simulink model "power_V2G"  (R2020b)
settings: Solver=ode23tb  StartTime=0.0  StopTime=24*60*60  RelTol=5e-4  AbsTol=5e-3
PreLoadFcn:
  | % Load Data and Parameters used by the model:
  | load power_V2G.mat
  | to=0.1;
undefined symbols (not defined in the file): A, B, C, D1, Dd, Delta, Init, j, V2G
libraries: powerlib x47, simulink x19, powerlib_meascontrol x7, simulink_extras x6, spsDieselMotorModel x1, sps_avr x1, V2Glib x1
(part 2 of 2)

== system power_V2G/Wind Farm 4.5 MW/Avoid division by zero ==
  I : Inport
  Complex to Magnitude-Angle : ComplexToMagnitudeAngle
  Magnitude-Angle to Complex : MagnitudeAngleToComplex
  Saturation1 : Saturate  UpperLimit=inf  LowerLimit=1e-6
  O : Outport  VectorParamsAs1DForOutWhenUnconnected=off
  wires:
  I/1 -> Complex to Magnitude-Angle/1
  Saturation1/1 -> Magnitude-Angle to Complex/1
  Complex to Magnitude-Angle/1 -> Saturation1/1
  Magnitude-Angle to Complex/1 -> O/1
  Complex to Magnitude-Angle/2 -> Magnitude-Angle to Complex/2

== system power_V2G/Wind Farm 4.5 MW/Break Alg. Loop 1 ==
  In : Inport
  Complex to Real-Imag : ComplexToRealImag
  Real-Imag to Complex : RealImagToComplex
  imag : Subsystem  mask(Transfer Function with Initial Outputs){N=[1], D=[to  1], Y0=0, U0=0}
      mask prompts: N "Numerator:"; D "Denominator:"; Y0 "Initial output:"; U0 "Initial input:"
      mask help: Vector expressions for numerator, and denominator. Coefficients are in descending powers of s.
      mask init:
      | [A,B,C,Dd]=tf2ss(N,D);if (isempty(Y0));[m,n]=size(A);X0=zeros(1,m); end; if (isempty(U0));[m,p]=size(B);U0=zeros(1,p);end;X0=getxo(A,B,C,Dd,U0,Y0,0);
      mask Help: Specify the initial output for the transfer function.  An optimization routine attempts to determine the appropriate initial states so that the specified initial output is achieved.  For more details, see the m-file getxo.m
      mask Display: dpoly(N,D,'s')
  real : Subsystem  mask(Transfer Function with Initial Outputs){N=[1], D=[to 1], Y0=0, U0=0}
      mask prompts: N "Numerator:"; D "Denominator:"; Y0 "Initial output:"; U0 "Initial input:"
      mask help: Vector expressions for numerator, and denominator. Coefficients are in descending powers of s.
      mask init:
      | [A,B,C,Dd]=tf2ss(N,D);if (isempty(Y0));[m,n]=size(A);X0=zeros(1,m); end; if (isempty(U0));[m,p]=size(B);U0=zeros(1,p);end;X0=getxo(A,B,C,Dd,U0,Y0,0);
      mask Help: Specify the initial output for the transfer function.  An optimization routine attempts to determine the appropriate initial states so that the specified initial output is achieved.  For more details, see the m-file getxo.m
      mask Display: dpoly(N,D,'s')
  Out : Outport  VectorParamsAs1DForOutWhenUnconnected=off
  wires:
  In/1 -> Complex to Real-Imag/1
  Real-Imag to Complex/1 -> Out/1
  real/1(Out1) -> Real-Imag to Complex/1
  imag/1(Out1) -> Real-Imag to Complex/2
  Complex to Real-Imag/2 -> imag/1(In1)
  Complex to Real-Imag/1 -> real/1(In1)

== system power_V2G/Wind Farm 4.5 MW/Wind farm control ==
  "wind " : Inport
  Compare To Constant : simulink/Logic and Bit Operations/Compare To Constant  relop=>=  const=maxwind-0.1  OutDataTypeStr=boolean  ZeroCross=off
  Compare To Constant1 : simulink/Logic and Bit Operations/Compare To Constant  relop=<=  const=nomwind  OutDataTypeStr=boolean  ZeroCross=off
  Constant1 : Constant  Value=0
  Constant2 : Constant  Value=9
  Logical Operator1 : Logic  Operator=NOT  AllPortsSameDT=off  OutDataTypeStr=boolean
  Manual Switch : ManualSwitch
  Rate Limiter2 : RateLimiter  RisingSlewLimit=1e4  FallingSlewLimit=-1e4  SampleTimeMode=inherited
  S-R Flip-Flop : simulink_extras/Flip Flops/S-R Flip-Flop  initial_condition=0
  Switch : Switch  Threshold=0.5  ZeroCross=off
  Terminator : Terminator
  Wind : Outport  VectorParamsAs1DForOutWhenUnconnected=off
  wires:
  "wind "/1 -> Switch/1, Compare To Constant/1, Compare To Constant1/1
  Constant1/1 -> Switch/3
  Logical Operator1/1 -> Switch/2
  S-R Flip-Flop/1 -> Logical Operator1/1
  Compare To Constant1/1 -> S-R Flip-Flop/2
  Compare To Constant/1 -> S-R Flip-Flop/1
  S-R Flip-Flop/2 -> Terminator/1
  Switch/1 -> Manual Switch/1
  Manual Switch/1 -> Rate Limiter2/1
  Constant2/1 -> Manual Switch/2
  Rate Limiter2/1 -> Wind/1

== system power_V2G/PV Farm 8 MW/Break Alg. Loop 1/imag ==
  In1 : Inport
  State Space : StateSpace  A=A  B=B  C=C  D=Dd  InitialCondition=X0
  Out1 : Outport  InitialOutput=0  VectorParamsAs1DForOutWhenUnconnected=off
  wires:
  State Space/1 -> Out1/1
  In1/1 -> State Space/1

== system power_V2G/PV Farm 8 MW/Break Alg. Loop 1/real ==
  In1 : Inport
  State Space : StateSpace  A=A  B=B  C=C  D=Dd  InitialCondition=X0
  Out1 : Outport  InitialOutput=0  VectorParamsAs1DForOutWhenUnconnected=off
  wires:
  State Space/1 -> Out1/1
  In1/1 -> State Space/1

== system power_V2G/Residential Load = 10 MW, PF=0.15 Industrial Load = 0.16 MVA /Residential Load/Avoid division by zero ==
  I : Inport
  Complex to Magnitude-Angle : ComplexToMagnitudeAngle
  Magnitude-Angle to Complex : MagnitudeAngleToComplex
  Saturation1 : Saturate  UpperLimit=inf  LowerLimit=1e-6
  O : Outport  VectorParamsAs1DForOutWhenUnconnected=off
  wires:
  I/1 -> Complex to Magnitude-Angle/1
  Saturation1/1 -> Magnitude-Angle to Complex/1
  Complex to Magnitude-Angle/1 -> Saturation1/1
  Magnitude-Angle to Complex/1 -> O/1
  Complex to Magnitude-Angle/2 -> Magnitude-Angle to Complex/2

== system power_V2G/Residential Load = 10 MW, PF=0.15 Industrial Load = 0.16 MVA /Residential Load/Break Alg. Loop 1 ==
  In : Inport
  Complex to Real-Imag : ComplexToRealImag
  Real-Imag to Complex : RealImagToComplex
  imag : Subsystem  mask(Transfer Function with Initial Outputs){N=[1], D=[to  1], Y0=0, U0=0}
      mask prompts: N "Numerator:"; D "Denominator:"; Y0 "Initial output:"; U0 "Initial input:"
      mask help: Vector expressions for numerator, and denominator. Coefficients are in descending powers of s.
      mask init:
      | [A,B,C,Dd]=tf2ss(N,D);if (isempty(Y0));[m,n]=size(A);X0=zeros(1,m); end; if (isempty(U0));[m,p]=size(B);U0=zeros(1,p);end;X0=getxo(A,B,C,Dd,U0,Y0,0);
      mask Help: Specify the initial output for the transfer function.  An optimization routine attempts to determine the appropriate initial states so that the specified initial output is achieved.  For more details, see the m-file getxo.m
      mask Display: dpoly(N,D,'s')
  real : Subsystem  mask(Transfer Function with Initial Outputs){N=[1], D=[to 1], Y0=0, U0=0}
      mask prompts: N "Numerator:"; D "Denominator:"; Y0 "Initial output:"; U0 "Initial input:"
      mask help: Vector expressions for numerator, and denominator. Coefficients are in descending powers of s.
      mask init:
      | [A,B,C,Dd]=tf2ss(N,D);if (isempty(Y0));[m,n]=size(A);X0=zeros(1,m); end; if (isempty(U0));[m,p]=size(B);U0=zeros(1,p);end;X0=getxo(A,B,C,Dd,U0,Y0,0);
      mask Help: Specify the initial output for the transfer function.  An optimization routine attempts to determine the appropriate initial states so that the specified initial output is achieved.  For more details, see the m-file getxo.m
      mask Display: dpoly(N,D,'s')
  Out : Outport  VectorParamsAs1DForOutWhenUnconnected=off
  wires:
  Complex to Real-Imag/1 -> real/1(In1)
  Complex to Real-Imag/2 -> imag/1(In1)
  In/1 -> Complex to Real-Imag/1
  Real-Imag to Complex/1 -> Out/1
  real/1(Out1) -> Real-Imag to Complex/1
  imag/1(Out1) -> Real-Imag to Complex/2

== system power_V2G/Residential Load = 10 MW, PF=0.15 Industrial Load = 0.16 MVA /Residential Load/Load ==
  1 : Constant
  Add : Sum
  Clock : Clock
  Constant : Constant
  Constant1 : Constant  Value=15/24
  Divide : Product  Inputs=*/
  Manual Switch : ManualSwitch
  Mux : Mux  Inputs=2
  P nom : Constant  Value=-nomPower*1e6
  Power consumption : Lookup_n-D  NumberOfTableDimensions=1  BreakpointsForDimension1=[1:timestep/60:24]  BeginIndexSearchUsingPreviousIndexResult=on  Table=datas  InternalRulePriority=Speed  RndMeth=Simplest  InputSameDT=on
  Power factor : Constant  Value=PF^2
  Product : Product
  Product1 : Product
  Scope : Scope
  Second-->Hour : Gain  Gain=1/(60*60)
  Sqrt : Sqrt  SaturateOnIntegerOverflow=on
  Sum : Sum  Inputs=-+
  PQ : Outport  VectorParamsAs1DForOutWhenUnconnected=off
  wires:
  Constant/1 -> Add/2
  1/1 -> Sum/1, Divide/1
  Second-->Hour/1 -> Add/1
  Sum/1 -> Sqrt/1
  Power factor/1 -> Divide/2
  Add/1 -> Power consumption/1
  P nom/1 -> Product/2
  Clock/1 -> Second-->Hour/1
  Sqrt/1 -> Product1/2
  Product/1 -> Product1/1, Mux/1
  Divide/1 -> Sum/2
  Product1/1 -> Mux/2
  Power consumption/1 -> Manual Switch/1
  Manual Switch/1 -> Product/1
  Constant1/1 -> Manual Switch/2
  Mux/1 -> Scope/1, PQ/1

== system power_V2G/V2G 4 MW (100x40 kW)/Car profiles/Car profile 1 ==
  Add : Sum
  Charger control : Subsystem
  Clock : Clock
  Constant : Constant
  Plug state : Lookup_n-D  NumberOfTableDimensions=1  BreakpointsForDimension1=[1:24]  BeginIndexSearchUsingPreviousIndexResult=on  Table="[1 1 1 1 1 1 0 0 1 1 1 1 1 1 1 1 0 0 1 1 1 1  1 1]"  InterpMethod=Flat  InternalRulePriority=Speed  RndMeth=Simplest  InputSameDT=on
  Rate Limiter : RateLimiter  RisingSlewLimit=1e4  FallingSlewLimit=-1e4  SampleTimeMode=inherited
  Rate Limiter1 : RateLimiter  RisingSlewLimit=1e4  FallingSlewLimit=-1e4  SampleTimeMode=inherited
  SOC initialization : Lookup_n-D  NumberOfTableDimensions=1  BreakpointsForDimension1=[1:24]  BeginIndexSearchUsingPreviousIndexResult=on  Table=[0.9 0.9 0.9 0.9 0.9 0.9 -1 0.8 0.8 0.9 0.9 0.9 0.9 0.9 0.9 0.9 -1 0.8 0.8 0.9 0.9 0.9 0.9 0.9]  InterpMethod=Flat  InternalRulePriority=Speed  RndMeth=Simplest  InputSameDT=on
  Second-->Hour : Gain  Gain=1/(60*60)
  State of charge : Subsystem
  "Regulation mode " : Outport  VectorParamsAs1DForOutWhenUnconnected=off
  "Charge mode " : Outport  Port=2  VectorParamsAs1DForOutWhenUnconnected=off
  wires:
  Constant/1 -> Add/2
  Second-->Hour/1 -> Add/1
  Clock/1 -> Second-->Hour/1
  Add/1 -> SOC initialization/1, Plug state/1
  State of charge/1(SE%) -> Charger control/1(SE%)
  Charger control/1("Charge mode ") -> State of charge/1(charge), "Charge mode "/1
  Charger control/2("Regulation mode ") -> "Regulation mode "/1
  SOC initialization/1 -> Rate Limiter/1
  Plug state/1 -> Rate Limiter1/1
  Rate Limiter/1 -> State of charge/2(SOC)
  Rate Limiter1/1 -> State of charge/3(Plug), Charger control/2("Plug ")

== system power_V2G/V2G 4 MW (100x40 kW)/Car profiles/Car profile 2 ==
  Add1 : Sum
  Charger control : Subsystem
  Clock1 : Clock
  Constant1 : Constant
  Plug state : Lookup_n-D  NumberOfTableDimensions=1  BreakpointsForDimension1=[1:24]  BeginIndexSearchUsingPreviousIndexResult=on  Table="[1 1 1 1 1 1 0 0 0 0 0 0 0 0 0 0 0 0 1 1 1 1  1 1]"  InterpMethod=Flat  InternalRulePriority=Speed  RndMeth=Simplest  InputSameDT=on
  Rate Limiter2 : RateLimiter  RisingSlewLimit=1e4  FallingSlewLimit=-1e4  SampleTimeMode=inherited
  Rate Limiter3 : RateLimiter  RisingSlewLimit=1e4  FallingSlewLimit=-1e4  SampleTimeMode=inherited
  SOC initialization : Lookup_n-D  NumberOfTableDimensions=1  BreakpointsForDimension1=[1:24]  BeginIndexSearchUsingPreviousIndexResult=on  Table=[0.9 0.9 0.9 0.9 0.9 0.9 -1 0.8 0.8 0.9 0.9 0.9 0.9 0.9 0.9 0.9 -1 0.8 0.6 0.9 0.9 0.9 0.9 0.9]  InterpMethod=Flat  InternalRulePriority=Speed  RndMeth=Simplest  InputSameDT=on
  Second-->Hour1 : Gain  Gain=1/(60*60)
  State of charge : Subsystem
  "Regulation mode " : Outport  VectorParamsAs1DForOutWhenUnconnected=off
  "Charge mode " : Outport  Port=2  VectorParamsAs1DForOutWhenUnconnected=off
  wires:
  Constant1/1 -> Add1/2
  Second-->Hour1/1 -> Add1/1
  Clock1/1 -> Second-->Hour1/1
  Add1/1 -> Plug state/1, SOC initialization/1
  State of charge/1(SE%) -> Charger control/1(SE%)
  Charger control/1("Charge mode ") -> State of charge/1(charge), "Charge mode "/1
  Charger control/2("Regulation mode ") -> "Regulation mode "/1
  SOC initialization/1 -> Rate Limiter2/1
  Plug state/1 -> Rate Limiter3/1
  Rate Limiter2/1 -> State of charge/2(SOC)
  Rate Limiter3/1 -> State of charge/3(Plug), Charger control/2("Plug ")

== system power_V2G/V2G 4 MW (100x40 kW)/Car profiles/Car profile 3 ==
  Add1 : Sum
  Charger control : Subsystem
  Clock1 : Clock
  Constant1 : Constant
  Plug state : Lookup_n-D  NumberOfTableDimensions=1  BreakpointsForDimension1=[1:24]  BeginIndexSearchUsingPreviousIndexResult=on  Table="[1 1 1 1 1 0 0 0 1 1 1 1 1 1 1 1 0 0 0 1 1 1  1 1]"  InterpMethod=Flat  InternalRulePriority=Speed  RndMeth=Simplest  InputSameDT=on
  Rate Limiter2 : RateLimiter  RisingSlewLimit=1e4  FallingSlewLimit=-1e4  SampleTimeMode=inherited
  Rate Limiter3 : RateLimiter  RisingSlewLimit=1e4  FallingSlewLimit=-1e4  SampleTimeMode=inherited
  SOC initialization : Lookup_n-D  NumberOfTableDimensions=1  BreakpointsForDimension1=[1:24]  BeginIndexSearchUsingPreviousIndexResult=on  Table=[0.9 0.9 0.9 0.9 0.9 -1 -1 0.7 0.7 0.9 0.9 0.9 0.9 0.9 0.9 0.9 -1 0.8 0.7 0.9 0.9 0.9 0.9 0.9]  InterpMethod=Flat  InternalRulePriority=Speed  RndMeth=Simplest  InputSameDT=on
  Second-->Hour1 : Gain  Gain=1/(60*60)
  State of charge : Subsystem
  "Regulation mode " : Outport  VectorParamsAs1DForOutWhenUnconnected=off
  "Charge mode " : Outport  Port=2  VectorParamsAs1DForOutWhenUnconnected=off
  wires:
  Constant1/1 -> Add1/2
  Second-->Hour1/1 -> Add1/1
  Clock1/1 -> Second-->Hour1/1
  Add1/1 -> Plug state/1, SOC initialization/1
  Charger control/1("Charge mode ") -> State of charge/1(charge), "Charge mode "/1
  Charger control/2("Regulation mode ") -> "Regulation mode "/1
  SOC initialization/1 -> Rate Limiter2/1
  Plug state/1 -> Rate Limiter3/1
  Rate Limiter2/1 -> State of charge/2(SOC)
  Rate Limiter3/1 -> State of charge/3(Plug), Charger control/2("Plug ")
  State of charge/1(SE%) -> Charger control/1(SE%)

== system power_V2G/V2G 4 MW (100x40 kW)/Car profiles/Car profile 4 ==
  Add1 : Sum
  Charger control : Subsystem
  Clock1 : Clock
  Constant1 : Constant
  Plug state : Lookup_n-D  NumberOfTableDimensions=1  BreakpointsForDimension1=[1:24]  BeginIndexSearchUsingPreviousIndexResult=on  Table="[1 1 1 1 1 1 1 1 1 1 1 1 1 1 1 1 1 1 1 1 1 1  1 1]"  InterpMethod=Flat  InternalRulePriority=Speed  RndMeth=Simplest  InputSameDT=on
  Rate Limiter2 : RateLimiter  RisingSlewLimit=1e4  FallingSlewLimit=-1e4  SampleTimeMode=inherited
  Rate Limiter3 : RateLimiter  RisingSlewLimit=1e4  FallingSlewLimit=-1e4  SampleTimeMode=inherited
  SOC initialization : Lookup_n-D  NumberOfTableDimensions=1  BreakpointsForDimension1=[1:24]  BeginIndexSearchUsingPreviousIndexResult=on  Table=[0.9 0.9 0.9 0.9 0.9 0.9 0.8 0.8 0.8 0.9 0.9 0.9 0.9 0.9 0.9 0.9 0.8 0.8 0.8 0.9 0.9 0.9 0.9 0.9]  InterpMethod=Flat  InternalRulePriority=Speed  RndMeth=Simplest  InputSameDT=on
  Second-->Hour1 : Gain  Gain=1/(60*60)
  State of charge : Subsystem
  "Regulation mode " : Outport  VectorParamsAs1DForOutWhenUnconnected=off
  "Charge mode " : Outport  Port=2  VectorParamsAs1DForOutWhenUnconnected=off
  wires:
  Constant1/1 -> Add1/2
  Second-->Hour1/1 -> Add1/1
  Clock1/1 -> Second-->Hour1/1
  Add1/1 -> Plug state/1, SOC initialization/1
  State of charge/1(SE%) -> Charger control/1(SE%)
  Charger control/1("Charge mode ") -> State of charge/1(charge), "Charge mode "/1
  Charger control/2("Regulation mode ") -> "Regulation mode "/1
  SOC initialization/1 -> Rate Limiter2/1
  Plug state/1 -> Rate Limiter3/1
  Rate Limiter2/1 -> State of charge/2(SOC)
  Rate Limiter3/1 -> State of charge/3(Plug), Charger control/2("Plug ")

== system power_V2G/V2G 4 MW (100x40 kW)/Car profiles/Car profile 5 ==
  Add : Sum
  Charger control : Subsystem
  Clock : Clock
  Constant : Constant
  Plug state : Lookup_n-D  NumberOfTableDimensions=1  BreakpointsForDimension1=[1:24]  BeginIndexSearchUsingPreviousIndexResult=on  Table="[0 0 0 0 1 1 1 1 1 1 1 1 1 1 1 1 1 1 1 1 0 0  0 0]"  InterpMethod=Flat  InternalRulePriority=Speed  RndMeth=Simplest  InputSameDT=on
  Rate Limiter : RateLimiter  RisingSlewLimit=1e4  FallingSlewLimit=-1e4  SampleTimeMode=inherited
  Rate Limiter1 : RateLimiter  RisingSlewLimit=1e4  FallingSlewLimit=-1e4  SampleTimeMode=inherited
  SOC initialization : Lookup_n-D  NumberOfTableDimensions=1  BreakpointsForDimension1=[1:24]  BeginIndexSearchUsingPreviousIndexResult=on  Table=[-1 0.9 0.7 0.7 0.7 0.8 0.8 0.8 0.8 0.8 0.9 0.9 0.9 0.9 0.9 0.9 0.8 0.8 0.8 0.9 -1 0.9 0.9 0.9]  InterpMethod=Flat  InternalRulePriority=Speed  RndMeth=Simplest  InputSameDT=on
  Second-->Hour : Gain  Gain=1/(60*60)
  State of charge : Subsystem
  "Regulation mode " : Outport  VectorParamsAs1DForOutWhenUnconnected=off
  "Charge mode " : Outport  Port=2  VectorParamsAs1DForOutWhenUnconnected=off
  wires:
  SOC initialization/1 -> Rate Limiter1/1
  Plug state/1 -> Rate Limiter/1
  Charger control/2("Regulation mode ") -> "Regulation mode "/1
  Charger control/1("Charge mode ") -> "Charge mode "/1, State of charge/1(charge)
  Add/1 -> Plug state/1, SOC initialization/1
  Clock/1 -> Second-->Hour/1
  Second-->Hour/1 -> Add/1
  Constant/1 -> Add/2
  State of charge/1(SE%) -> Charger control/1(SE%)
  Rate Limiter/1 -> Charger control/2("Plug "), State of charge/3(Plug)
  Rate Limiter1/1 -> State of charge/2(SOC)

== system power_V2G/V2G 4 MW (100x40 kW)/Charge load/Avoid division by zero ==
  I : Inport
  Complex to Magnitude-Angle : ComplexToMagnitudeAngle
  Magnitude-Angle to Complex : MagnitudeAngleToComplex
  Saturation1 : Saturate  UpperLimit=inf  LowerLimit=1e-6
  O : Outport  VectorParamsAs1DForOutWhenUnconnected=off
  wires:
  I/1 -> Complex to Magnitude-Angle/1
  Saturation1/1 -> Magnitude-Angle to Complex/1
  Complex to Magnitude-Angle/1 -> Saturation1/1
  Magnitude-Angle to Complex/1 -> O/1
  Complex to Magnitude-Angle/2 -> Magnitude-Angle to Complex/2

== system power_V2G/V2G 4 MW (100x40 kW)/Charge load/Break Alg. Loop 2 ==
  In : Inport
  Complex to Real-Imag : ComplexToRealImag
  Real-Imag to Complex : RealImagToComplex
  imag : Subsystem  mask(Transfer Function with Initial Outputs){N=[1], D=[to  1], Y0=0, U0=0}
      mask prompts: N "Numerator:"; D "Denominator:"; Y0 "Initial output:"; U0 "Initial input:"
      mask help: Vector expressions for numerator, and denominator. Coefficients are in descending powers of s.
      mask init:
      | [A,B,C,Dd]=tf2ss(N,D);if (isempty(Y0));[m,n]=size(A);X0=zeros(1,m); end; if (isempty(U0));[m,p]=size(B);U0=zeros(1,p);end;X0=getxo(A,B,C,Dd,U0,Y0,0);
      mask Help: Specify the initial output for the transfer function.  An optimization routine attempts to determine the appropriate initial states so that the specified initial output is achieved.  For more details, see the m-file getxo.m
      mask Display: dpoly(N,D,'s')
  real : Subsystem  mask(Transfer Function with Initial Outputs){N=[1], D=[to 1], Y0=0, U0=0}
      mask prompts: N "Numerator:"; D "Denominator:"; Y0 "Initial output:"; U0 "Initial input:"
      mask help: Vector expressions for numerator, and denominator. Coefficients are in descending powers of s.
      mask init:
      | [A,B,C,Dd]=tf2ss(N,D);if (isempty(Y0));[m,n]=size(A);X0=zeros(1,m); end; if (isempty(U0));[m,p]=size(B);U0=zeros(1,p);end;X0=getxo(A,B,C,Dd,U0,Y0,0);
      mask Help: Specify the initial output for the transfer function.  An optimization routine attempts to determine the appropriate initial states so that the specified initial output is achieved.  For more details, see the m-file getxo.m
      mask Display: dpoly(N,D,'s')
  Out : Outport  VectorParamsAs1DForOutWhenUnconnected=off
  wires:
  Complex to Real-Imag/1 -> real/1(In1)
  Complex to Real-Imag/2 -> imag/1(In1)
  In/1 -> Complex to Real-Imag/1
  Real-Imag to Complex/1 -> Out/1
  real/1(Out1) -> Real-Imag to Complex/1
  imag/1(Out1) -> Real-Imag to Complex/2

== system power_V2G/V2G 4 MW (100x40 kW)/Grid regulation/Grid regulation ocntrol ==
  Pmax reg : Inport
  Clock : Clock
  Compare To Constant : simulink/Logic and Bit Operations/Compare To Constant  relop=>=  const=5e-4  OutDataTypeStr=boolean  ZeroCross=off
  Compare To Constant1 : simulink/Logic and Bit Operations/Compare To Constant  relop=<=  const=-5e-4  OutDataTypeStr=boolean  ZeroCross=off
  Compare To Constant2 : simulink/Logic and Bit Operations/Compare To Constant  relop=>  const=1  OutDataTypeStr=boolean  ZeroCross=off
  Derivative : Derivative
  Gain : Gain  Gain=regGain(2)*1e6
  Gain1 : Gain  Gain=regGain(1)*1e6
  Gain2 : Gain  Gain=-1
  Integrator Limited : Integrator  ExternalReset=falling  UpperSaturationLimit=1e6  LowerSaturationLimit=-1e6
  Logical Operator : Logic  Operator=OR  AllPortsSameDT=off  OutDataTypeStr=boolean
  Logical Operator1 : Logic  AllPortsSameDT=off  OutDataTypeStr=boolean
  Mux : Mux  Inputs=2
  Q : Constant  Value=0
  Q1 : Constant  Value=0
  Saturation Dynamic : simulink/Discontinuities/Saturation Dynamic  OutMin=[]  OutMax=[]  OutDataTypeStr=Inherit: Same as second input  OutDataType=fixdt(1, 16)  OutScaling=2^-10  DoSatur=off
  Sum : Sum  Inputs=|+-
  Sum1 : Sum  Inputs=|++
  Switch : Switch  Threshold=0.5  ZeroCross=off
  wref : Constant
  PQ : Outport  VectorParamsAs1DForOutWhenUnconnected=off
  wires:
  Compare To Constant2/1 -> Logical Operator1/2
  Clock/1 -> Compare To Constant2/1
  Logical Operator/1 -> Logical Operator1/1
  Gain2/1 -> Saturation Dynamic/3
  Pmax reg/1 -> Saturation Dynamic/1, Gain2/1
  Integrator Limited/1 -> Saturation Dynamic/2
  Compare To Constant1/1 -> Logical Operator/2
  Compare To Constant/1 -> Logical Operator/1
  Sum/1 -> Switch/1, Compare To Constant/1, Compare To Constant1/1
  Switch/1 -> Derivative/1, Gain/1
  Gain/1 -> Sum1/2
  Gain1/1 -> Sum1/1
  Derivative/1 -> Gain1/1
  Sum1/1 -> Integrator Limited/1
  Q1/1 -> Switch/3
  [wm] -> Sum/2
  wref/1 -> Sum/1
  Q/1 -> Mux/2
  Mux/1 -> PQ/1
  Logical Operator1/1 -> Integrator Limited/2, Switch/2
  Saturation Dynamic/1 -> Mux/1

== system power_V2G/V2G 4 MW (100x40 kW)/Grid regulation/Grid regulation power  generation ==
  note: V1= 1/3(Vab -a^2*Vbc)
  note: S = 3* ( V * I') / 2
  note: Ia= I1
  note: Ib= a^2*I1
  "PQ " : Inport
  Add : Sum  Inputs=+-
  Avoid division by zero : Subsystem
  Break Alg. Loop 1 : Subsystem
  Conj1 : Math  Operator=conj  SignedPower=on  SaturateOnIntegerOverflow=on
  Demux : Demux  Outputs=2
  Product : Product  Inputs=/*  InputSameDT=on  SaturateOnIntegerOverflow=on  OutDataTypeStr=Inherit: Same as first input
  Real-Imag to Complex : RealImagToComplex
  a^2 : Gain  Gain=exp(-j*2*pi/3)  SaturateOnIntegerOverflow=on  OutDataTypeStr=Inherit: Same as input  ParamDataTypeStr=Inherit: Same as input
  "a^2 " : Gain  Gain=exp(-j*2*pi/3)  SaturateOnIntegerOverflow=on  OutDataTypeStr=Inherit: Same as input  ParamDataTypeStr=Inherit: Same as input
  a^3 : Gain  Gain=1/3  SaturateOnIntegerOverflow=on  OutDataTypeStr=Inherit: Same as input  ParamDataTypeStr=Inherit: Same as input
  a^4 : Gain  Gain=2/3  SaturateOnIntegerOverflow=on  OutDataTypeStr=Inherit: Same as input  ParamDataTypeStr=Inherit: Same as input
  tag scope: Ia1=global, Ib1=global
  wires:
  Real-Imag to Complex/1 -> Product/2
  Product/1 -> a^4/1  "I1"
  Avoid division by zero/1(O) -> Product/1  "V1"
  Conj1/1 -> Break Alg. Loop 1/1(In)
  a^3/1 -> Avoid division by zero/1(I)
  Add/1 -> a^3/1
  [Vab1] -> Add/1
  [Vbc1] -> "a^2 "/1
  "a^2 "/1 -> Add/2
  a^4/1 -> Conj1/1
  Break Alg. Loop 1/1(Out) -> [Ia1], a^2/1
  Demux/1 -> Real-Imag to Complex/1
  Demux/2 -> Real-Imag to Complex/2
  "PQ "/1 -> Demux/1
  a^2/1 -> [Ib1]

== system power_V2G/Wind Farm 4.5 MW/Break Alg. Loop 1/imag ==
  In1 : Inport
  State Space : StateSpace  A=A  B=B  C=C  D=Dd  InitialCondition=X0
  Out1 : Outport  InitialOutput=0  VectorParamsAs1DForOutWhenUnconnected=off
  wires:
  State Space/1 -> Out1/1
  In1/1 -> State Space/1

== system power_V2G/Wind Farm 4.5 MW/Break Alg. Loop 1/real ==
  In1 : Inport
  State Space : StateSpace  A=A  B=B  C=C  D=Dd  InitialCondition=X0
  Out1 : Outport  InitialOutput=0  VectorParamsAs1DForOutWhenUnconnected=off
  wires:
  State Space/1 -> Out1/1
  In1/1 -> State Space/1

== system power_V2G/Residential Load = 10 MW, PF=0.15 Industrial Load = 0.16 MVA /Residential Load/Break Alg. Loop 1/imag ==
  In1 : Inport
  State Space : StateSpace  A=A  B=B  C=C  D=Dd  InitialCondition=X0
  Out1 : Outport  InitialOutput=0  VectorParamsAs1DForOutWhenUnconnected=off
  wires:
  State Space/1 -> Out1/1
  In1/1 -> State Space/1

== system power_V2G/Residential Load = 10 MW, PF=0.15 Industrial Load = 0.16 MVA /Residential Load/Break Alg. Loop 1/real ==
  In1 : Inport
  State Space : StateSpace  A=A  B=B  C=C  D=Dd  InitialCondition=X0
  Out1 : Outport  InitialOutput=0  VectorParamsAs1DForOutWhenUnconnected=off
  wires:
  State Space/1 -> Out1/1
  In1/1 -> State Space/1

== system power_V2G/V2G 4 MW (100x40 kW)/Car profiles/Car profile 1/Charger control ==
  SE% : Inport
  "Plug " : Inport  Port=2
  Compare To Constant : simulink/Logic and Bit Operations/Compare To Constant  relop=<=  const=85  OutDataTypeStr=boolean  ZeroCross=off
  Compare To Constant1 : simulink/Logic and Bit Operations/Compare To Constant  relop=>=  const=95  OutDataTypeStr=boolean  ZeroCross=off
  Logical Operator : Logic  AllPortsSameDT=off  OutDataTypeStr=boolean
  Logical Operator1 : Logic  Operator=NOT  AllPortsSameDT=off  OutDataTypeStr=boolean
  Logical Operator2 : Logic  AllPortsSameDT=off  OutDataTypeStr=boolean
  S-R Flip-Flop : simulink_extras/Flip Flops/S-R Flip-Flop  initial_condition=0
  Terminator : Terminator
  "Charge mode " : Outport  VectorParamsAs1DForOutWhenUnconnected=off
  "Regulation mode " : Outport  Port=2  VectorParamsAs1DForOutWhenUnconnected=off
  wires:
  SE%/1 -> Compare To Constant/1, Compare To Constant1/1
  Compare To Constant/1 -> S-R Flip-Flop/1
  Compare To Constant1/1 -> S-R Flip-Flop/2
  "Plug "/1 -> Logical Operator2/2, Logical Operator/2
  S-R Flip-Flop/1 -> Logical Operator/1, Logical Operator1/1
  Logical Operator/1 -> "Charge mode "/1
  Logical Operator2/1 -> "Regulation mode "/1
  Logical Operator1/1 -> Logical Operator2/1
  S-R Flip-Flop/2 -> Terminator/1

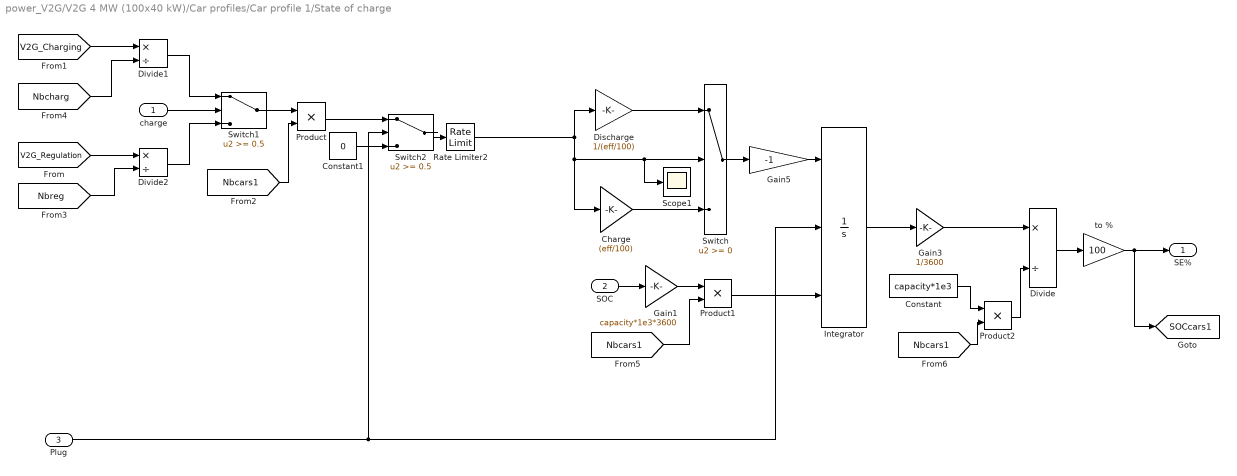
== system power_V2G/V2G 4 MW (100x40 kW)/Car profiles/Car profile 1/State of charge ==
  charge : Inport
  SOC : Inport  Port=2
  Plug : Inport  Port=3
  Charge : Gain  Gain=(eff/100)
  Constant : Constant  Value=capacity*1e3
  Constant1 : Constant  Value=0
  Discharge : Gain  Gain=1/(eff/100)
  Divide : Product  Inputs=*/
  Divide1 : Product  Inputs=*/
  Divide2 : Product  Inputs=*/
  Gain1 : Gain  Gain=capacity*1e3*3600
  Gain3 : Gain  Gain=1/3600
  Gain5 : Gain  Gain=-1
  Integrator : Integrator  ExternalReset=either  InitialConditionSource=external  InitialCondition=Init*850e3*3600
  Product : Product
  Product1 : Product
  Product2 : Product
  Rate Limiter2 : RateLimiter  RisingSlewLimit=1e4  FallingSlewLimit=-1e4  SampleTimeMode=inherited
  Scope1 : Scope
  Switch : Switch  ZeroCross=off
  Switch1 : Switch  Threshold=0.5  ZeroCross=off
  Switch2 : Switch  Threshold=0.5  ZeroCross=off
  to % : Gain  Gain=100
  SE% : Outport  VectorParamsAs1DForOutWhenUnconnected=off
  tag scope: SOCcars1=global
  wires:
  Discharge/1 -> Switch/1
  Charge/1 -> Switch/3
  Switch/1 -> Gain5/1
  Gain5/1 -> Integrator/1
  Integrator/1 -> Gain3/1
  Divide/1 -> to %/1
  Gain3/1 -> Divide/1
  to %/1 -> [SOCcars1], SE%/1
  Plug/1 -> Integrator/2, Switch2/2
  SOC/1 -> Gain1/1
  charge/1 -> Switch1/2
  Rate Limiter2/1 -> Discharge/1, Charge/1, Scope1/1, Switch/2
  [V2G_Charging] -> Divide1/1
  [Nbreg] -> Divide2/2
  [V2G_Regulation] -> Divide2/1
  [Nbcharg] -> Divide1/2
  [Nbcars1] -> Product/2
  Divide2/1 -> Switch1/3
  Constant1/1 -> Switch2/3
  Switch2/1 -> Rate Limiter2/1
  [Nbcars1] -> Product1/2
  Gain1/1 -> Product1/1
  Product1/1 -> Integrator/3
  Product2/1 -> Divide/2
  [Nbcars1] -> Product2/2
  Constant/1 -> Product2/1
  Divide1/1 -> Switch1/1
  Switch1/1 -> Product/1
  Product/1 -> Switch2/1

== system power_V2G/V2G 4 MW (100x40 kW)/Car profiles/Car profile 2/Charger control ==
  SE% : Inport
  "Plug " : Inport  Port=2
  Compare To Constant : simulink/Logic and Bit Operations/Compare To Constant  relop=<=  const=85  OutDataTypeStr=boolean  ZeroCross=off
  Compare To Constant1 : simulink/Logic and Bit Operations/Compare To Constant  relop=>=  const=95  OutDataTypeStr=boolean  ZeroCross=off
  Logical Operator : Logic  AllPortsSameDT=off  OutDataTypeStr=boolean
  Logical Operator1 : Logic  Operator=NOT  AllPortsSameDT=off  OutDataTypeStr=boolean
  Logical Operator2 : Logic  AllPortsSameDT=off  OutDataTypeStr=boolean
  S-R Flip-Flop : simulink_extras/Flip Flops/S-R Flip-Flop  initial_condition=0
  Terminator : Terminator
  "Charge mode " : Outport  VectorParamsAs1DForOutWhenUnconnected=off
  "Regulation mode " : Outport  Port=2  VectorParamsAs1DForOutWhenUnconnected=off
  wires:
  SE%/1 -> Compare To Constant/1, Compare To Constant1/1
  Compare To Constant/1 -> S-R Flip-Flop/1
  Compare To Constant1/1 -> S-R Flip-Flop/2
  "Plug "/1 -> Logical Operator2/2, Logical Operator/2
  S-R Flip-Flop/1 -> Logical Operator/1, Logical Operator1/1
  Logical Operator/1 -> "Charge mode "/1
  Logical Operator2/1 -> "Regulation mode "/1
  Logical Operator1/1 -> Logical Operator2/1
  S-R Flip-Flop/2 -> Terminator/1

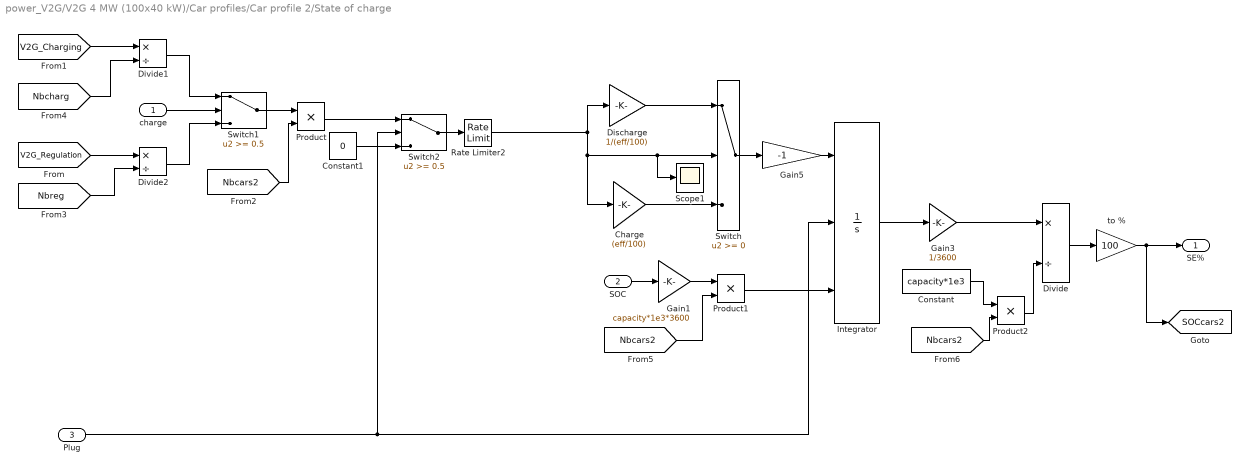
== system power_V2G/V2G 4 MW (100x40 kW)/Car profiles/Car profile 2/State of charge ==
  charge : Inport
  SOC : Inport  Port=2
  Plug : Inport  Port=3
  Charge : Gain  Gain=(eff/100)
  Constant : Constant  Value=capacity*1e3
  Constant1 : Constant  Value=0
  Discharge : Gain  Gain=1/(eff/100)
  Divide : Product  Inputs=*/
  Divide1 : Product  Inputs=*/
  Divide2 : Product  Inputs=*/
  Gain1 : Gain  Gain=capacity*1e3*3600
  Gain3 : Gain  Gain=1/3600
  Gain5 : Gain  Gain=-1
  Integrator : Integrator  ExternalReset=either  InitialConditionSource=external  InitialCondition=Init*850e3*3600
  Product : Product
  Product1 : Product
  Product2 : Product
  Rate Limiter2 : RateLimiter  RisingSlewLimit=1e4  FallingSlewLimit=-1e4  SampleTimeMode=inherited
  Scope1 : Scope
  Switch : Switch  ZeroCross=off
  Switch1 : Switch  Threshold=0.5  ZeroCross=off
  Switch2 : Switch  Threshold=0.5  ZeroCross=off
  to % : Gain  Gain=100
  SE% : Outport  VectorParamsAs1DForOutWhenUnconnected=off
  tag scope: SOCcars2=global
  wires:
  Discharge/1 -> Switch/1
  Charge/1 -> Switch/3
  Switch/1 -> Gain5/1
  Gain5/1 -> Integrator/1
  Integrator/1 -> Gain3/1
  Divide/1 -> to %/1
  Gain3/1 -> Divide/1
  to %/1 -> [SOCcars2], SE%/1
  SOC/1 -> Gain1/1
  Rate Limiter2/1 -> Discharge/1, Charge/1, Scope1/1, Switch/2
  [Nbcars2] -> Product1/2
  Gain1/1 -> Product1/1
  Product1/1 -> Integrator/3
  Product2/1 -> Divide/2
  [Nbcars2] -> Product2/2
  Constant/1 -> Product2/1
  Switch1/1 -> Product/1
  Divide1/1 -> Switch1/1
  [V2G_Charging] -> Divide1/1
  Product/1 -> Switch2/1
  [Nbreg] -> Divide2/2
  charge/1 -> Switch1/2
  [Nbcars2] -> Product/2
  Divide2/1 -> Switch1/3
  Constant1/1 -> Switch2/3
  [V2G_Regulation] -> Divide2/1
  Plug/1 -> Integrator/2, Switch2/2
  [Nbcharg] -> Divide1/2
  Switch2/1 -> Rate Limiter2/1

== system power_V2G/V2G 4 MW (100x40 kW)/Car profiles/Car profile 3/Charger control ==
  SE% : Inport
  "Plug " : Inport  Port=2
  Compare To Constant : simulink/Logic and Bit Operations/Compare To Constant  relop=<=  const=85  OutDataTypeStr=boolean  ZeroCross=off
  Compare To Constant1 : simulink/Logic and Bit Operations/Compare To Constant  relop=>=  const=95  OutDataTypeStr=boolean  ZeroCross=off
  Logical Operator : Logic  AllPortsSameDT=off  OutDataTypeStr=boolean
  Logical Operator1 : Logic  Operator=NOT  AllPortsSameDT=off  OutDataTypeStr=boolean
  Logical Operator2 : Logic  AllPortsSameDT=off  OutDataTypeStr=boolean
  S-R Flip-Flop : simulink_extras/Flip Flops/S-R Flip-Flop  initial_condition=0
  Terminator : Terminator
  "Charge mode " : Outport  VectorParamsAs1DForOutWhenUnconnected=off
  "Regulation mode " : Outport  Port=2  VectorParamsAs1DForOutWhenUnconnected=off
  wires:
  SE%/1 -> Compare To Constant/1, Compare To Constant1/1
  Compare To Constant/1 -> S-R Flip-Flop/1
  Compare To Constant1/1 -> S-R Flip-Flop/2
  "Plug "/1 -> Logical Operator2/2, Logical Operator/2
  S-R Flip-Flop/1 -> Logical Operator/1, Logical Operator1/1
  Logical Operator/1 -> "Charge mode "/1
  Logical Operator2/1 -> "Regulation mode "/1
  Logical Operator1/1 -> Logical Operator2/1
  S-R Flip-Flop/2 -> Terminator/1

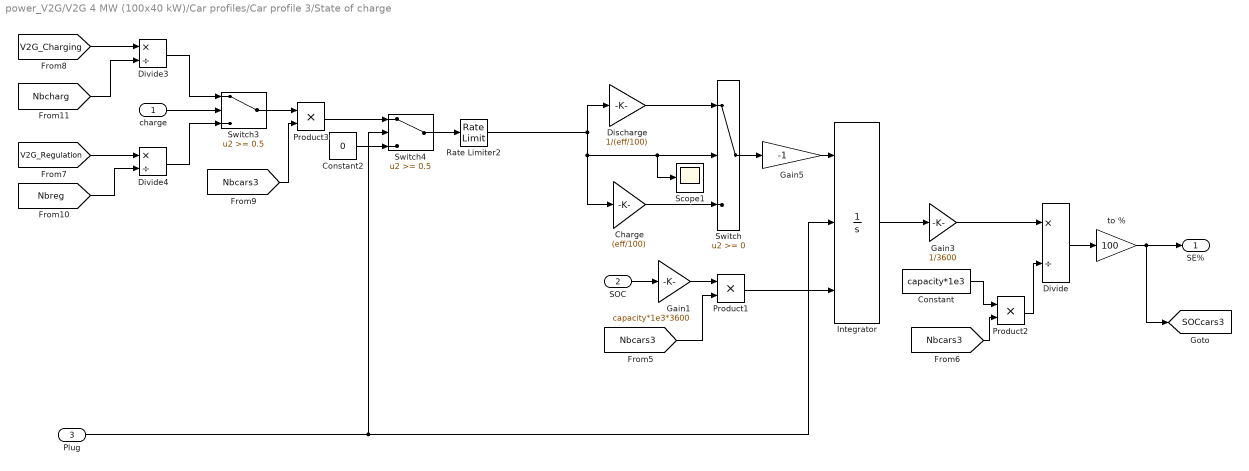
== system power_V2G/V2G 4 MW (100x40 kW)/Car profiles/Car profile 3/State of charge ==
  charge : Inport
  SOC : Inport  Port=2
  Plug : Inport  Port=3
  Charge : Gain  Gain=(eff/100)
  Constant : Constant  Value=capacity*1e3
  Constant2 : Constant  Value=0
  Discharge : Gain  Gain=1/(eff/100)
  Divide : Product  Inputs=*/
  Divide3 : Product  Inputs=*/
  Divide4 : Product  Inputs=*/
  Gain1 : Gain  Gain=capacity*1e3*3600
  Gain3 : Gain  Gain=1/3600
  Gain5 : Gain  Gain=-1
  Integrator : Integrator  ExternalReset=either  InitialConditionSource=external  InitialCondition=Init*850e3*3600
  Product1 : Product
  Product2 : Product
  Product3 : Product
  Rate Limiter2 : RateLimiter  RisingSlewLimit=1e4  FallingSlewLimit=-1e4  SampleTimeMode=inherited
  Scope1 : Scope
  Switch : Switch  ZeroCross=off
  Switch3 : Switch  Threshold=0.5  ZeroCross=off
  Switch4 : Switch  Threshold=0.5  ZeroCross=off
  to % : Gain  Gain=100
  SE% : Outport  VectorParamsAs1DForOutWhenUnconnected=off
  tag scope: SOCcars3=global
  wires:
  Discharge/1 -> Switch/1
  Charge/1 -> Switch/3
  Switch/1 -> Gain5/1
  Gain5/1 -> Integrator/1
  Integrator/1 -> Gain3/1
  Divide/1 -> to %/1
  Gain3/1 -> Divide/1
  to %/1 -> [SOCcars3], SE%/1
  SOC/1 -> Gain1/1
  Rate Limiter2/1 -> Discharge/1, Charge/1, Scope1/1, Switch/2
  Switch4/1 -> Rate Limiter2/1
  [Nbcars3] -> Product1/2
  Gain1/1 -> Product1/1
  Product1/1 -> Integrator/3
  Product2/1 -> Divide/2
  [Nbcars3] -> Product2/2
  Constant/1 -> Product2/1
  Switch3/1 -> Product3/1
  Divide3/1 -> Switch3/1
  [V2G_Charging] -> Divide3/1
  Product3/1 -> Switch4/1
  [Nbreg] -> Divide4/2
  charge/1 -> Switch3/2
  [Nbcars3] -> Product3/2
  Divide4/1 -> Switch3/3
  Constant2/1 -> Switch4/3
  [V2G_Regulation] -> Divide4/1
  Plug/1 -> Switch4/2, Integrator/2
  [Nbcharg] -> Divide3/2

== system power_V2G/V2G 4 MW (100x40 kW)/Car profiles/Car profile 4/Charger control ==
  SE% : Inport
  "Plug " : Inport  Port=2
  Compare To Constant : simulink/Logic and Bit Operations/Compare To Constant  relop=<=  const=85  OutDataTypeStr=boolean  ZeroCross=off
  Compare To Constant1 : simulink/Logic and Bit Operations/Compare To Constant  relop=>=  const=95  OutDataTypeStr=boolean  ZeroCross=off
  Logical Operator : Logic  AllPortsSameDT=off  OutDataTypeStr=boolean
  Logical Operator1 : Logic  Operator=NOT  AllPortsSameDT=off  OutDataTypeStr=boolean
  Logical Operator2 : Logic  AllPortsSameDT=off  OutDataTypeStr=boolean
  S-R Flip-Flop : simulink_extras/Flip Flops/S-R Flip-Flop  initial_condition=0
  Terminator : Terminator
  "Charge mode " : Outport  VectorParamsAs1DForOutWhenUnconnected=off
  "Regulation mode " : Outport  Port=2  VectorParamsAs1DForOutWhenUnconnected=off
  wires:
  SE%/1 -> Compare To Constant/1, Compare To Constant1/1
  Compare To Constant/1 -> S-R Flip-Flop/1
  Compare To Constant1/1 -> S-R Flip-Flop/2
  "Plug "/1 -> Logical Operator2/2, Logical Operator/2
  S-R Flip-Flop/1 -> Logical Operator/1, Logical Operator1/1
  Logical Operator/1 -> "Charge mode "/1
  Logical Operator2/1 -> "Regulation mode "/1
  Logical Operator1/1 -> Logical Operator2/1
  S-R Flip-Flop/2 -> Terminator/1

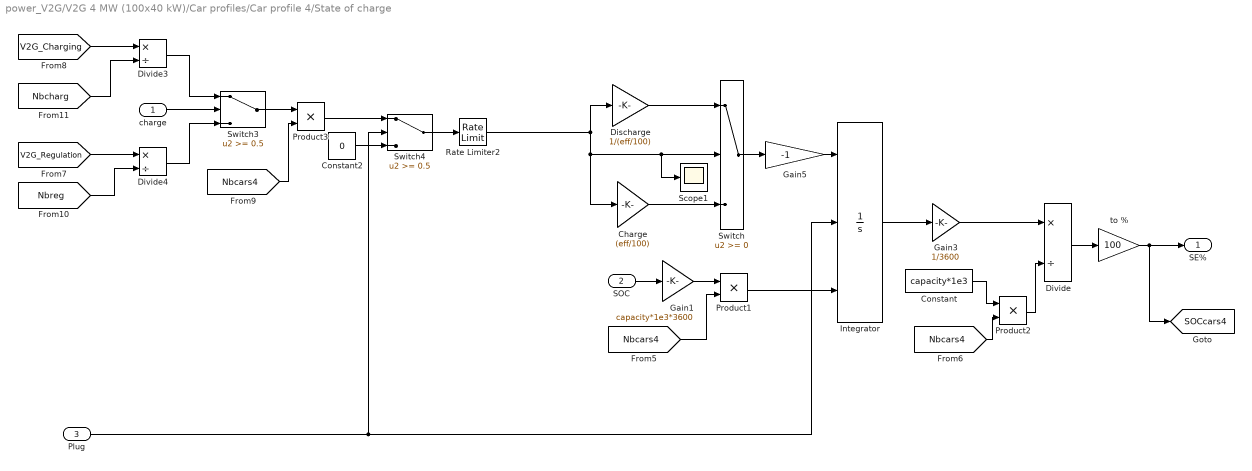
== system power_V2G/V2G 4 MW (100x40 kW)/Car profiles/Car profile 4/State of charge ==
  charge : Inport
  SOC : Inport  Port=2
  Plug : Inport  Port=3
  Charge : Gain  Gain=(eff/100)
  Constant : Constant  Value=capacity*1e3
  Constant2 : Constant  Value=0
  Discharge : Gain  Gain=1/(eff/100)
  Divide : Product  Inputs=*/
  Divide3 : Product  Inputs=*/
  Divide4 : Product  Inputs=*/
  Gain1 : Gain  Gain=capacity*1e3*3600
  Gain3 : Gain  Gain=1/3600
  Gain5 : Gain  Gain=-1
  Integrator : Integrator  ExternalReset=either  InitialConditionSource=external  InitialCondition=Init*850e3*3600
  Product1 : Product
  Product2 : Product
  Product3 : Product
  Rate Limiter2 : RateLimiter  RisingSlewLimit=1e4  FallingSlewLimit=-1e4  SampleTimeMode=inherited
  Scope1 : Scope
  Switch : Switch  ZeroCross=off
  Switch3 : Switch  Threshold=0.5  ZeroCross=off
  Switch4 : Switch  Threshold=0.5  ZeroCross=off
  to % : Gain  Gain=100
  SE% : Outport  VectorParamsAs1DForOutWhenUnconnected=off
  tag scope: SOCcars4=global
  wires:
  Discharge/1 -> Switch/1
  Charge/1 -> Switch/3
  Switch/1 -> Gain5/1
  Gain5/1 -> Integrator/1
  Integrator/1 -> Gain3/1
  Divide/1 -> to %/1
  Gain3/1 -> Divide/1
  to %/1 -> [SOCcars4], SE%/1
  SOC/1 -> Gain1/1
  Rate Limiter2/1 -> Discharge/1, Charge/1, Scope1/1, Switch/2
  [Nbcars4] -> Product1/2
  Gain1/1 -> Product1/1
  Product1/1 -> Integrator/3
  Product2/1 -> Divide/2
  [Nbcars4] -> Product2/2
  Constant/1 -> Product2/1
  [Nbcars4] -> Product3/2
  [Nbcharg] -> Divide3/2
  [V2G_Regulation] -> Divide4/1
  Divide4/1 -> Switch3/3
  charge/1 -> Switch3/2
  Constant2/1 -> Switch4/3
  Product3/1 -> Switch4/1
  [V2G_Charging] -> Divide3/1
  [Nbreg] -> Divide4/2
  Divide3/1 -> Switch3/1
  Switch4/1 -> Rate Limiter2/1
  Switch3/1 -> Product3/1
  Plug/1 -> Switch4/2, Integrator/2

== system power_V2G/V2G 4 MW (100x40 kW)/Car profiles/Car profile 5/Charger control ==
  SE% : Inport
  "Plug " : Inport  Port=2
  Compare To Constant : simulink/Logic and Bit Operations/Compare To Constant  relop=<=  const=85  OutDataTypeStr=boolean
  Compare To Constant1 : simulink/Logic and Bit Operations/Compare To Constant  relop=>=  const=95  OutDataTypeStr=boolean
  Logical Operator : Logic  AllPortsSameDT=off  OutDataTypeStr=boolean
  Logical Operator1 : Logic  Operator=NOT  AllPortsSameDT=off  OutDataTypeStr=boolean
  Logical Operator2 : Logic  AllPortsSameDT=off  OutDataTypeStr=boolean
  S-R Flip-Flop : simulink_extras/Flip Flops/S-R Flip-Flop  initial_condition=0
  Terminator : Terminator
  "Charge mode " : Outport  VectorParamsAs1DForOutWhenUnconnected=off
  "Regulation mode " : Outport  Port=2  VectorParamsAs1DForOutWhenUnconnected=off
  wires:
  S-R Flip-Flop/2 -> Terminator/1
  Logical Operator1/1 -> Logical Operator2/1
  Logical Operator2/1 -> "Regulation mode "/1
  Logical Operator/1 -> "Charge mode "/1
  S-R Flip-Flop/1 -> Logical Operator/1, Logical Operator1/1
  "Plug "/1 -> Logical Operator/2, Logical Operator2/2
  Compare To Constant1/1 -> S-R Flip-Flop/2
  Compare To Constant/1 -> S-R Flip-Flop/1
  SE%/1 -> Compare To Constant/1, Compare To Constant1/1

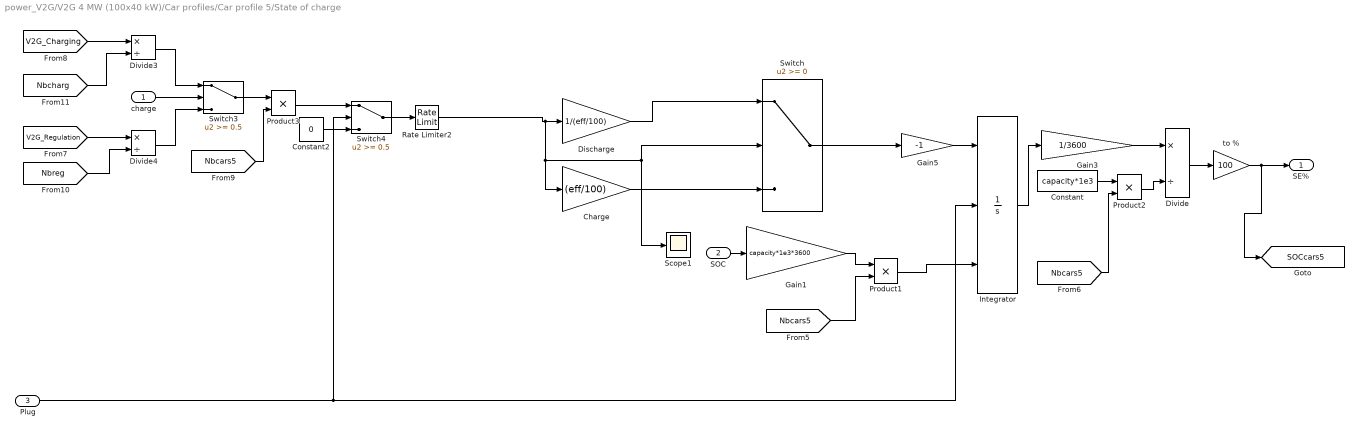
== system power_V2G/V2G 4 MW (100x40 kW)/Car profiles/Car profile 5/State of charge ==
  charge : Inport
  SOC : Inport  Port=2
  Plug : Inport  Port=3
  Charge : Gain  Gain=(eff/100)
  Constant : Constant  Value=capacity*1e3
  Constant2 : Constant  Value=0
  Discharge : Gain  Gain=1/(eff/100)
  Divide : Product  Inputs=*/
  Divide3 : Product  Inputs=*/
  Divide4 : Product  Inputs=*/
  Gain1 : Gain  Gain=capacity*1e3*3600
  Gain3 : Gain  Gain=1/3600
  Gain5 : Gain  Gain=-1
  Integrator : Integrator  ExternalReset=either  InitialConditionSource=external  InitialCondition=Init*850e3*3600
  Product1 : Product
  Product2 : Product
  Product3 : Product
  Rate Limiter2 : RateLimiter  RisingSlewLimit=1e4  FallingSlewLimit=-1e4  SampleTimeMode=inherited
  Scope1 : Scope
  Switch : Switch  ZeroCross=off
  Switch3 : Switch  Threshold=0.5  ZeroCross=off
  Switch4 : Switch  Threshold=0.5  ZeroCross=off
  to % : Gain  Gain=100
  SE% : Outport  VectorParamsAs1DForOutWhenUnconnected=off
  tag scope: SOCcars5=global
  wires:
  Product2/1 -> Divide/2
  Constant/1 -> Product2/1
  [Nbcars5] -> Product2/2
  Product1/1 -> Integrator/3
  [Nbcars5] -> Product1/2
  Gain1/1 -> Product1/1
  Rate Limiter2/1 -> Discharge/1, Charge/1, Switch/2, Scope1/1
  SOC/1 -> Gain1/1
  to %/1 -> SE%/1, [SOCcars5]
  Gain3/1 -> Divide/1
  Divide/1 -> to %/1
  Integrator/1 -> Gain3/1
  Gain5/1 -> Integrator/1
  Switch/1 -> Gain5/1
  Charge/1 -> Switch/3
  Discharge/1 -> Switch/1
  [Nbcars5] -> Product3/2
  [Nbcharg] -> Divide3/2
  [V2G_Regulation] -> Divide4/1
  Divide4/1 -> Switch3/3
  charge/1 -> Switch3/2
  Constant2/1 -> Switch4/3
  Product3/1 -> Switch4/1
  [V2G_Charging] -> Divide3/1
  [Nbreg] -> Divide4/2
  Divide3/1 -> Switch3/1
  Switch4/1 -> Rate Limiter2/1
  Switch3/1 -> Product3/1
  Plug/1 -> Switch4/2, Integrator/2

== system power_V2G/V2G 4 MW (100x40 kW)/Charge load/Break Alg. Loop 2/imag ==
  In1 : Inport
  State Space : StateSpace  A=A  B=B  C=C  D=Dd  InitialCondition=X0
  Out1 : Outport  InitialOutput=0  VectorParamsAs1DForOutWhenUnconnected=off
  wires:
  State Space/1 -> Out1/1
  In1/1 -> State Space/1

== system power_V2G/V2G 4 MW (100x40 kW)/Charge load/Break Alg. Loop 2/real ==
  In1 : Inport
  State Space : StateSpace  A=A  B=B  C=C  D=Dd  InitialCondition=X0
  Out1 : Outport  InitialOutput=0  VectorParamsAs1DForOutWhenUnconnected=off
  wires:
  State Space/1 -> Out1/1
  In1/1 -> State Space/1

== system power_V2G/V2G 4 MW (100x40 kW)/Grid regulation/Grid regulation power  generation/Avoid division by zero ==
  I : Inport
  Complex to Magnitude-Angle : ComplexToMagnitudeAngle
  Magnitude-Angle to Complex : MagnitudeAngleToComplex
  Saturation1 : Saturate  UpperLimit=inf  LowerLimit=1e-6
  O : Outport  VectorParamsAs1DForOutWhenUnconnected=off
  wires:
  I/1 -> Complex to Magnitude-Angle/1
  Saturation1/1 -> Magnitude-Angle to Complex/1
  Complex to Magnitude-Angle/1 -> Saturation1/1
  Magnitude-Angle to Complex/1 -> O/1
  Complex to Magnitude-Angle/2 -> Magnitude-Angle to Complex/2

== system power_V2G/V2G 4 MW (100x40 kW)/Grid regulation/Grid regulation power  generation/Break Alg. Loop 1 ==
  In : Inport
  Complex to Real-Imag : ComplexToRealImag
  Real-Imag to Complex : RealImagToComplex
  imag : Subsystem  mask(Transfer Function with Initial Outputs){N=[1], D=[to  1], Y0=0, U0=0}
      mask prompts: N "Numerator:"; D "Denominator:"; Y0 "Initial output:"; U0 "Initial input:"
      mask help: Vector expressions for numerator, and denominator. Coefficients are in descending powers of s.
      mask init:
      | [A,B,C,Dd]=tf2ss(N,D);if (isempty(Y0));[m,n]=size(A);X0=zeros(1,m); end; if (isempty(U0));[m,p]=size(B);U0=zeros(1,p);end;X0=getxo(A,B,C,Dd,U0,Y0,0);
      mask Help: Specify the initial output for the transfer function.  An optimization routine attempts to determine the appropriate initial states so that the specified initial output is achieved.  For more details, see the m-file getxo.m
      mask Display: dpoly(N,D,'s')
  real : Subsystem  mask(Transfer Function with Initial Outputs){N=[1], D=[to 1], Y0=0, U0=0}
      mask prompts: N "Numerator:"; D "Denominator:"; Y0 "Initial output:"; U0 "Initial input:"
      mask help: Vector expressions for numerator, and denominator. Coefficients are in descending powers of s.
      mask init:
      | [A,B,C,Dd]=tf2ss(N,D);if (isempty(Y0));[m,n]=size(A);X0=zeros(1,m); end; if (isempty(U0));[m,p]=size(B);U0=zeros(1,p);end;X0=getxo(A,B,C,Dd,U0,Y0,0);
      mask Help: Specify the initial output for the transfer function.  An optimization routine attempts to determine the appropriate initial states so that the specified initial output is achieved.  For more details, see the m-file getxo.m
      mask Display: dpoly(N,D,'s')
  Out : Outport  VectorParamsAs1DForOutWhenUnconnected=off
  wires:
  Complex to Real-Imag/1 -> real/1(In1)
  Complex to Real-Imag/2 -> imag/1(In1)
  In/1 -> Complex to Real-Imag/1
  Real-Imag to Complex/1 -> Out/1
  real/1(Out1) -> Real-Imag to Complex/1
  imag/1(Out1) -> Real-Imag to Complex/2

== system power_V2G/V2G 4 MW (100x40 kW)/Grid regulation/Grid regulation power  generation/Break Alg. Loop 1/imag ==
  In1 : Inport
  State Space : StateSpace  A=A  B=B  C=C  D=Dd  InitialCondition=X0
  Out1 : Outport  InitialOutput=0  VectorParamsAs1DForOutWhenUnconnected=off
  wires:
  State Space/1 -> Out1/1
  In1/1 -> State Space/1

== system power_V2G/V2G 4 MW (100x40 kW)/Grid regulation/Grid regulation power  generation/Break Alg. Loop 1/real ==
  In1 : Inport
  State Space : StateSpace  A=A  B=B  C=C  D=Dd  InitialCondition=X0
  Out1 : Outport  InitialOutput=0  VectorParamsAs1DForOutWhenUnconnected=off
  wires:
  State Space/1 -> Out1/1
  In1/1 -> State Space/1
